simulink model "mode_lame_a"  (R2020a)
settings: Solver=VariableStepAuto  StartTime=0.0  StopTime=2  RelTol=1e-3
settings Model: Creator=antoi  LastModifiedBy=SAGOU26

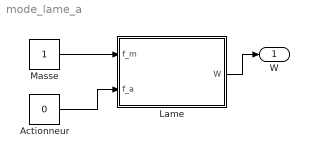
== system mode_lame_a ==
  Actionneur : Constant  Value=0
  Lame : MATLAB Function  TreatAsAtomicUnit=on
  Masse : Constant
  W : Outport
  wires:
  Masse/1 -> Lame/1(f_m)
  Actionneur/1 -> Lame/2(f_a)
  Lame/1(W) -> W/1

== matlab function mode_lame_a/Lame ==
  data: f_m input; W output; f_a input
function W  = fcn(f_m, f_a)
    X = load('Parameters.mat');
    
    % La force
    X.F(11) = f_a + f_m;
    
    %h = plot(X.x, X.w_init, X.x, X.w_new);
    xlabel("X [m]")
    ylabel("Déflexion [m]")
    ylim([-0.01,0.01])
    grid on

    
    for i = 3:X.nx-2
        
        %Équation différentielle résolue par Sam
        X.w_new(i) = (-X.coeff1*(X.w(i+2)-4*X.w(i+1)+6*X.w(i)-4*X.w(i-1)+X.w(i-2)) - X.coeff2*(-2*X.w(i)+X.w_old(i)) + X.coeff3*X.w(i) + X.F(i)/X.dx)*X.coeff4;

        %% Conditions limites 

        X.w_new(1:2) = 0;                 % Clampé à zero, position et dérivée nulle (le bout de la lame est fixe)

        X.w_new(end-1) = 2*X.w_new(end-2)-X.w_new(end-3);    % Libre au bout dérivées 2e et 3e nulles
        X.w_new(end) = 2*X.w_new(end-1)-X.w_new(end-2);
        
        %set(h(2), "Ydata", X.w_new);
        %drawnow
    end
     
    %% Préparation du prochain tour
    
    X.w_old = X.w;
    X.w = X.w_new;
    
    W = X.w(end);
end
